simulink model "aeropendulo"  (R2024b)
settings: Solver=VariableStepAuto  StartTime=0.0  StopTime=10.0  RelTol=1e-3
settings Model: Creator=ameli  LastModifiedBy=ameli

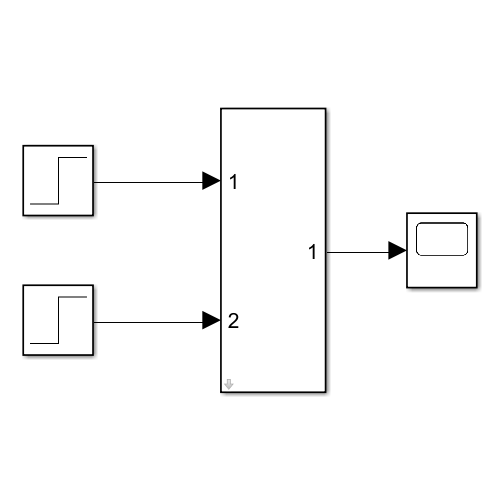
[thumbnail: Simulink's stored preview of the top-level diagram]
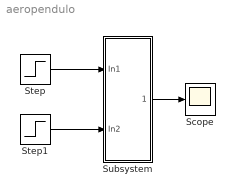
== system aeropendulo ==
  Scope : Scope
  Step : Step  Time=0  SampleTime=0
  Step1 : Step  Time=0  After=0  SampleTime=0
  Subsystem : Subsystem  mask{J=0.0333, l1=0.4, l2=0.2, m=0.5, g=9.81, d=0.1, b=0.1}
  wires:
  Step/1 -> Subsystem/1(In1)
  Step1/1 -> Subsystem/2(In2)
  Subsystem/1(Out1) -> Scope/1

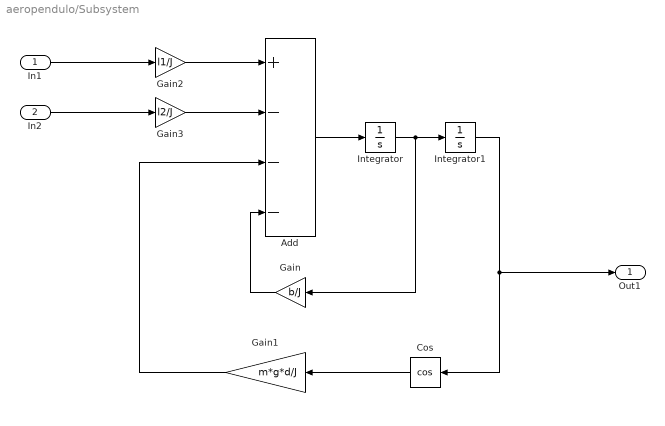
== system aeropendulo/Subsystem ==
  In1 : Inport
  In2 : Inport  Port=2
  Add : Sum  Inputs=+---
  Cos : Trigonometry  Operator=cos
  Gain : Gain  Gain=b/J
  Gain1 : Gain  Gain=m*g*d/J
  Gain2 : Gain  Gain=l1/J
  Gain3 : Gain  Gain=l2/J
  Integrator : Integrator
  Integrator1 : Integrator
  Out1 : Outport
  wires:
  Integrator/1 -> Gain/1, Integrator1/1
  Cos/1 -> Gain1/1
  Gain/1 -> Add/4
  Add/1 -> Integrator/1
  Integrator1/1 -> Out1/1, Cos/1
  Gain1/1 -> Add/3
  In1/1 -> Gain2/1
  Gain2/1 -> Add/1
  In2/1 -> Gain3/1
  Gain3/1 -> Add/2
